simulink model "AppMain"  (R2021a)
settings: Solver=FixedStepDiscrete  StartTime=0.0  StopTime=80  FixedStep=10e-3  RelTol=1e-3
PreLoadFcn:
  | AppMain_data
values from neighbouring files (symbols this model uses):
  CtrlConst = struct    [AppMain_data.m]
  TaskTimeBase = struct    [AppMain_data.m]
undefined symbols (not defined in the file or in its folder): Lock, Open, Short
libraries: simulink x27, lib1 x10
(part 3 of 3)

== matlab function AppMain/PwmInTargetSpeedEval/NormalState/PwmInSpeedCtrl/PwmInNotShort/DutyFilter/Enabled Subsystem/DutyFilter/DutyValid/BufDataSameFirstCnt ==
  data: buf input; samecnt output; tolerance input
function samecnt = BufDataSameFirstCnt(buf,tolerance)
if buf(1,1) >= tolerance
    min = buf(1,1) - tolerance;
else
    min = uint16(0);
end

max = buf(1,1) + tolerance;
if max > 1000
   max = uint16(1000); 
end

samecnt = uint16(1);
for i = 2:length(buf)
    if buf(i) >= min && buf(i) <= max
       samecnt = samecnt + 1; 
    end
end

== stateflow chart AppMain/PwmInTargetSpeedEval/NormalState/PwmInSpeedCtrl/PwmInNotShort/FreqValidJudge/FreqValidJudge ==
  state Invalid
    entry:
    Valid = false;
    ValidCnt = 1;
    Invalid -> (junction 37) [order 1] : {Valid = false;}
    (junction 37) -> (junction 38) [order 1] : [    (Freq <= FreqMax) ...
        | &&(Freq >= FreqMin)]
        | {ValidCnt = ValidCnt + 1;}
    (junction 37) -> (junction 38) [order 2] : {ValidCnt = 1;}
  state Valid
    entry:
    Valid = true;
    InvalidCnt = 1;
    Valid -> (junction 9) [order 1] : {Valid = true;}
    (junction 9) -> (junction 11) [order 1] : [ (Freq > FreqMax + FreqTolerance) ...
        | ||(Freq + FreqTolerance < FreqMin)]
        | {InvalidCnt = InvalidCnt + 1;}
    (junction 9) -> (junction 11) [order 2] : {InvalidCnt = 1; }
  (junction 56) -> Invalid
  (junction 54) -> (junction 56) [order 2]
  Valid -> Invalid [order 1] : [InvalidCnt >=FreqValidJudgeFilterTime]
  Invalid -> Valid [order 1] : [ValidCnt >=FreqValidJudgeFilterTime]
  (default) -> (junction 54)
  (junction 54) -> Valid [order 1] : [(Freq <= FreqMax + FreqTolerance) ...
      | &&(Freq + FreqTolerance >= FreqMin)]
  data: Freq input uint16; Valid output boolean =false; ValidCnt local uint16 =uint16(0); InvalidCnt local uint16 =uint16(0); FreqMin input uint16; FreqMax input uint16; FreqTolerance input uint16; FreqValidJudgeFilterTime input uint16

== stateflow chart AppMain/PwmInTargetSpeedEval/NormalState/PwmInSpeedCtrl/SpeedDelayOut/DelayOut ==
  state Delay
    Delay -> (junction 29) [order 1]
    (junction 29) -> (junction 30) [order 1] : [DelayCnt < DelayTHR]
        | {DelayCnt = DelayCnt + 1;
        | Out = OutLast;}
    (junction 29) -> (junction 31) [order 2]
    (junction 32) -> (junction 30)
    (junction 31) -> (junction 32) : {Out = In;}
  state Reset
    en:
    DelayCnt = 2;
    Out = OutLast;
  (default) -> Reset
  Reset -> Delay : [Rst == false]
  Delay -> Reset [order 1] : [Rst == true]
  data: DelayCnt local uint16 =uint16(0); In input int16; Out output int16 =int16(0); DelayTHR input uint16; Rst input boolean; OutLast input int16

== stateflow chart AppMain/MotorRestartAndFaultCnt/MotorFalutHandle/MotorFaultRecoverTimer/MotorRestartFSM ==
  state TimeCnt
    entry:
    TimeCnt = 1;
    RecoverEn = false;
    du:
    TimeCnt = TimeCnt + 1;
  state ReStart
    en:
    RecoverEn = true;
  (default) -> TimeCnt
  ReStart -> TimeCnt : [MotorRestartCompleted == true]
  TimeCnt -> ReStart : [TimeCnt >= TimeTHR && TimeTHR ~= 65535]
  data: TimeTHR input uint16; MotorRestartCompleted input boolean; TimeCnt local uint16 =uint16(0); RecoverEn output boolean =false

== stateflow chart AppMain/FeedBack/StateKeep ==
  state TrueState
    en:
    State = true;
    FalseTime = 0;
    du:
    State = true;
    TrueState -> (junction 20) [order 1]
    (junction 20) -> (junction 22) [order 1] : [TrueTime > 0]
        | {TrueTime = TrueTime -1;}
    (junction 20) -> (junction 30) [order 2]
    (junction 32) -> (junction 22)
    (junction 30) -> (junction 32)
  state FalseState
    en:
    State = false;
    TrueTime=TrueKeepTime;
    FalseTime=FalseKeepTime;
    du:
    State = false;
    FalseState -> (junction 25) [order 1]
    (junction 25) -> (junction 27) [order 1] : [FalseTime > 0]
        | {FalseTime = FalseTime - 1;}
    (junction 25) -> (junction 35) [order 2]
    (junction 37) -> (junction 27)
    (junction 35) -> (junction 37) [order 1] : [TrueTime == 0]
        | {TrueTime=TrueKeepTime;
        | FalseTime=FalseKeepTime;}
    (junction 35) -> (junction 45) [order 2]
    (junction 47) -> (junction 37)
    (junction 45) -> (junction 47)
  (default) -> (junction 40) : {TrueTime=TrueKeepTime;
      | FalseTime=FalseKeepTime;}
  (junction 40) -> (junction 42) [order 2]
  (junction 40) -> FalseState [order 1] : [FalseTime ~= 0]
  (junction 42) -> TrueState
  TrueState -> FalseState [order 1] : [(TrueTime <= 1) &&  (FalseKeepTime > 0)]
  FalseState -> TrueState [order 1] : [FalseTime <= 1 && TrueTime > 0]
  data: State output boolean; BusSateCnt local uint16; FalseTime local uint16 =uint16(65535); TrueTime local uint16 =uint16(65535); FalseKeepTime input uint16; TrueKeepTime input uint16
